simulink model "testFrame_rf_sbstm_detectStartUp"  (R2022b)
settings: Solver=FixedStepDiscrete  StartTime=0.0  StopTime=5  FixedStep=1  RelTol=1e-3
libraries: simulink x1
settings Model: Creator=unix  LastModifiedBy=unix

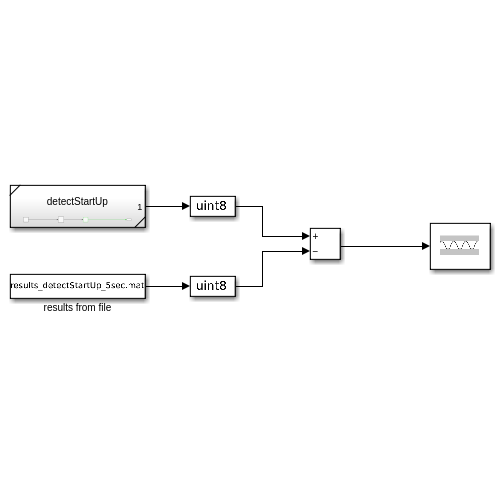
[thumbnail: Simulink's stored preview of the top-level diagram]
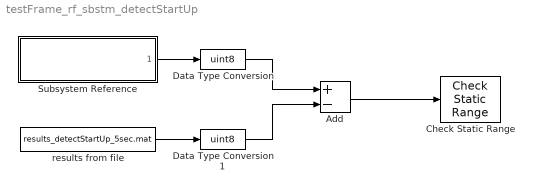
== system testFrame_rf_sbstm_detectStartUp ==
  Add : Sum  Inputs=+-  OutDataTypeStr=int8
  Check Static Range : simulink/Model Verification/Check  Static Range  Description=-0.1 <= u <= 0  max=0  max_included=on  min=-0.1  min_included=on  enabled=on  stopWhenAssertionFail=on  export=off  icon=graphic
  Data Type Conversion : DataTypeConversion  OutDataTypeStr=uint8  SaturateOnIntegerOverflow=off  RndMeth=Floor
  Data Type Conversion1 : DataTypeConversion  OutDataTypeStr=uint8  SaturateOnIntegerOverflow=off  RndMeth=Floor
  Subsystem Reference : Subsystem  ReferencedSubsystem=detectStartUp
  results from file : FromFile  FileName=results_detectStartUp_5sec.mat  SampleTime=0
  wires:
  Subsystem Reference/1 -> Data Type Conversion/1
  results from file/1 -> Data Type Conversion1/1
  Data Type Conversion/1 -> Add/1
  Add/1 -> Check Static Range/1
  Data Type Conversion1/1 -> Add/2
